simulink model "Counter"  (R2021a)
settings: Solver=FixedStepDiscrete  StartTime=0.0  StopTime=10.0  RelTol=1e-3  EnableMultiTasking=on
settings Model: Creator=top one  LastModifiedBy=top one
settings DataIOCC: ReturnWorkspaceOutputs=off
settings OptimizationCC: DefaultParameterBehavior=Inlined  InlineInvariantSignals=on  EnableMemcpy=off  LifeSpan=1  EfficientTunableParamExpr=on
settings DebuggingCC: UnderspecifiedInitializationDetection=Classic  MergeDetectMultiDrivingBlocksExec=none  SFMachineParentedDataDiag=warning  ArithmeticOperatorsInVariantConditions=warning
settings ModelReferenceCC: PropagateSignalLabelsOutOfModel=off
settings SFSimCC: MATLABDynamicMemAlloc=off  CustomCodeUndefinedFunction=UseInterfaceOnly
settings RTWCC: SystemTargetFile=ert.tlc  GenCodeOnly=on  TemplateMakefile=ert_default_tmf  GenerateReport=on  IncludeHyperlinkInReport=on  LaunchReport=on  GenerateTraceInfo=on  GenerateTraceReport=on  GenerateTraceReportSl=on  GenerateTraceReportSf=on  GenerateTraceReportEml=on
settings CodeAppCC: ForceParamTrailComments=on  IgnoreCustomStorageClasses=off  OperatorAnnotations=on  SimulinkDataObjDesc=on  SFDataObjDesc=on  MATLABFcnDesc=on  InsertBlockDesc=on  StateflowObjectComments=on  MATLABSourceComments=on
settings ERTTargetCC: MultiwordLength=2048  GenerateSampleERTMain=on  InlinedParameterPlacement=NonHierarchical  ERTCustomFileTemplate=example_file_process.tlc

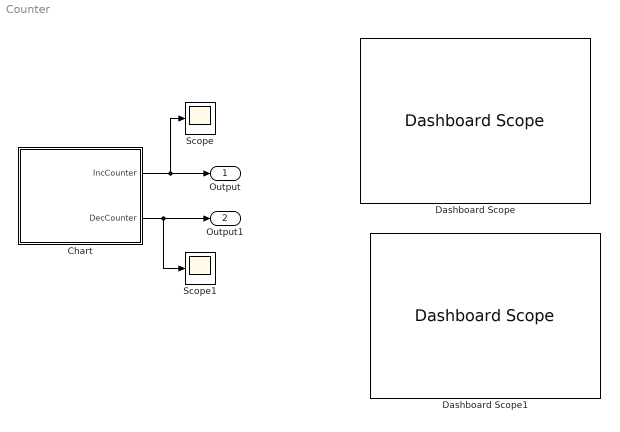
== system Counter ==
  Chart : Stateflow chart  TreatAsAtomicUnit=on
  Dashboard Scope : DashboardScope
  Dashboard Scope1 : DashboardScope
  Scope : Scope
  Scope1 : Scope
  Output : Outport
  Output1 : Outport  Port=2
  wires:
  Chart/1(IncCounter) -> Scope/1, Output/1
  Chart/2(DecCounter) -> Scope1/1, Output1/1

== stateflow chart Counter/Chart ==
  state Name
    IncCounter=0;
    DecCounter=10;
  state Name1
    IncCounter=IncCounter+1;
    DecCounter=DecCounter-1;
  (default) -> Name
  Name1 -> Name [order 1] : [IncCounter==10]
  Name -> Name1
  Name1 -> Name1 [order 2]
  data: IncCounter output =0; DecCounter output =10; index local
